simulink model "project_2"  (R2020a)
settings: Solver=ode45  StartTime=0.0  StopTime=10.0  MaxStep=0.01  RelTol=1e-3
values from neighbouring files (symbols this model uses):
  ic = 6    [project2.m]
libraries: simulink x1
settings Model: Creator=Matt  LastModifiedBy=Matt
settings DataIOCC: ReturnWorkspaceOutputs=off

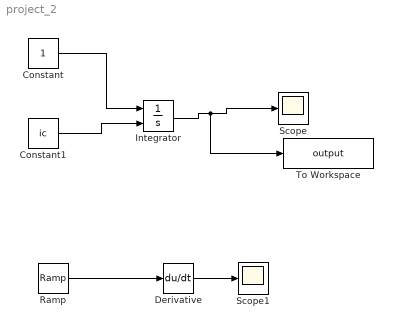
== system project_2 ==
  Constant : Constant
  Constant1 : Constant  Value=ic
  Derivative : Derivative
  Integrator : Integrator  InitialConditionSource=external  InitialCondition=2
  Ramp : simulink/Sources/Ramp  slope=1  start=0  InitialOutput=0
  Scope : Scope
  Scope1 : Scope
  To Workspace : ToWorkspace  VariableName=output  SampleTime=-1
  wires:
  Constant/1 -> Integrator/1
  Integrator/1 -> To Workspace/1, Scope/1
  Derivative/1 -> Scope1/1
  Ramp/1 -> Derivative/1
  Constant1/1 -> Integrator/2
